simulink model "rotor_simulink"  (R2022a)
settings: Solver=VariableStepAuto  StartTime=0.1  StopTime=60  FixedStep=sample_time/10  RelTol=1e-3
values from neighbouring files (symbols this model uses):
  I_eq = rotor.I + generator.I/gearbox.ratio^2    [parameters.m]
  K_opt = 0.5*(lambda_opt)^(-3)*rho*pi*rotor.R^5*cp_max    [rotor_test.m]
  lambda_vector = linspace(lambda_range(1), lambda_range(2), lambda_item)    [parameters.m]
  omega_rated = rated_values(2)    [parameters.m]
  pitch_range = deg2rad([-15 90])    [parameters.m]
  pitch_vector = linspace(pitch_range(1), pitch_range(2), pitch_item)    [parameters.m]
  rho = 1.225    [parameters.m]
  wind_speed = run_generated_wind_series(wind.mean(i),          wind.turbulence(i), wind_speed, stop_time)    [main.m]    (also in parameters.m = load('usim.dat'); rotor_test.m = WS(i))
undefined symbols (not defined in the file or in its folder): blade, gearbox, generator, lookup_cP, omega_r, rotor
settings Model: Creator=Niccolò  LastModifiedBy=Niccolò

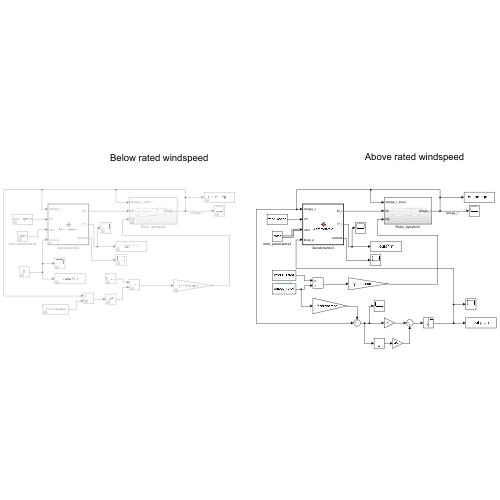
[thumbnail: Simulink's stored preview of the top-level diagram]
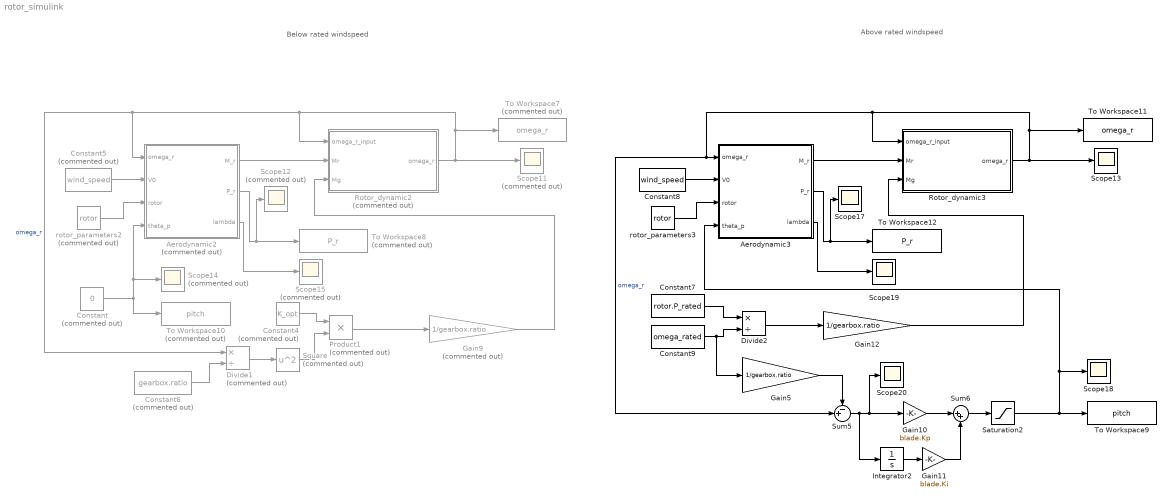
== system rotor_simulink ==
  note: Below rated windspeed
  note: Above rated windspeed
  Aerodynamic2 : MATLAB Function  Commented=on  TreatAsAtomicUnit=on
  Aerodynamic3 : MATLAB Function  TreatAsAtomicUnit=on
  Constant : Constant  Commented=on  Value=0
  Constant4 : Constant  Commented=on  Value=K_opt
  Constant5 : Constant  Commented=on  Value=wind_speed
  Constant6 : Constant  Commented=on  Value=gearbox.ratio
  Constant7 : Constant  Value=rotor.P_rated
  Constant8 : Constant  Value=wind_speed
  Constant9 : Constant  Value=omega_rated
  Divide1 : Product  Commented=on  Inputs=*/
  Divide2 : Product  Inputs=*/
  Gain10 : Gain  Gain=blade.Kp
  Gain11 : Gain  Gain=blade.Ki
  Gain12 : Gain  Gain=1/gearbox.ratio
  Gain5 : Gain  Gain=1/gearbox.ratio
  Gain9 : Gain  Commented=on  Gain=1/gearbox.ratio
  Integrator2 : Integrator
  Product1 : Product  Commented=on
  Rotor_dynamic2 : Subsystem  Commented=on
  Rotor_dynamic3 : Subsystem
  Saturation2 : Saturate  UpperLimit=30*pi/180  LowerLimit=pitch_range(1)
  Scope{11..12,14..15} (4 alike) : Scope  Commented=on
  Scope{13,17..20} (5 alike) : Scope
  Square : Math  Commented=on  Operator=square
  Sum5 : Sum  Inputs=-+|
  Sum6 : Sum  Inputs=|++
  To Workspace10 : ToWorkspace  Commented=on  VariableName=pitch  SaveFormat=Timeseries  SampleTime=-1
  To Workspace11 : ToWorkspace  VariableName=omega_r  SaveFormat=Timeseries  SampleTime=-1
  To Workspace12 : ToWorkspace  VariableName=P_r  SaveFormat=Timeseries  SampleTime=-1
  To Workspace7 : ToWorkspace  Commented=on  VariableName=omega_r  SaveFormat=Timeseries  SampleTime=-1
  To Workspace8 : ToWorkspace  Commented=on  VariableName=P_r  SaveFormat=Timeseries  SampleTime=-1
  To Workspace9 : ToWorkspace  VariableName=pitch  SaveFormat=Timeseries  SampleTime=-1
  rotor_parameters2 : Constant  Commented=on  Value=rotor  OutDataTypeStr=Bus: rotor_bus
  rotor_parameters3 : Constant  Value=rotor  OutDataTypeStr=Bus: rotor_bus
  wires:
  Rotor_dynamic2/1(omega_r) -> Scope11/1, To Workspace7/1, Rotor_dynamic2/1(omega_r_input), Divide1/1, Aerodynamic2/1(omega_r)  "omega_r"
  Constant5/1 -> Aerodynamic2/2(V0)
  Aerodynamic2/2(P_r) -> Scope12/1, To Workspace8/1
  Gain9/1 -> Rotor_dynamic2/3(Mg)
  Aerodynamic2/3(lambda) -> Scope15/1
  Aerodynamic2/1(M_r) -> Rotor_dynamic2/2(Mr)
  rotor_parameters2/1 -> Aerodynamic2/3(rotor)
  Saturation2/1 -> To Workspace9/1, Scope18/1, Aerodynamic3/4(theta_p)
  Sum6/1 -> Saturation2/1
  Constant7/1 -> Divide2/1
  Gain5/1 -> Sum5/1
  rotor_parameters3/1 -> Aerodynamic3/3(rotor)
  Integrator2/1 -> Gain11/1
  Aerodynamic3/1(M_r) -> Rotor_dynamic3/2(Mr)
  Aerodynamic3/3(lambda) -> Scope19/1
  Aerodynamic3/2(P_r) -> Scope17/1, To Workspace12/1
  Divide2/1 -> Gain12/1
  Gain10/1 -> Sum6/1
  Gain12/1 -> Rotor_dynamic3/3(Mg)
  Constant8/1 -> Aerodynamic3/2(V0)
  Constant9/1 -> Gain5/1, Divide2/2
  Sum5/1 -> Scope20/1, Gain10/1, Integrator2/1
  Gain11/1 -> Sum6/2
  Rotor_dynamic3/1(omega_r) -> Scope13/1, To Workspace11/1, Rotor_dynamic3/1(omega_r_input), Sum5/2, Aerodynamic3/1(omega_r)  "omega_r"
  Constant/1 -> Aerodynamic2/4(theta_p), Scope14/1, To Workspace10/1
  Constant4/1 -> Product1/1
  Divide1/1 -> Square/1
  Square/1 -> Product1/2
  Product1/1 -> Gain9/1
  Constant6/1 -> Divide1/2

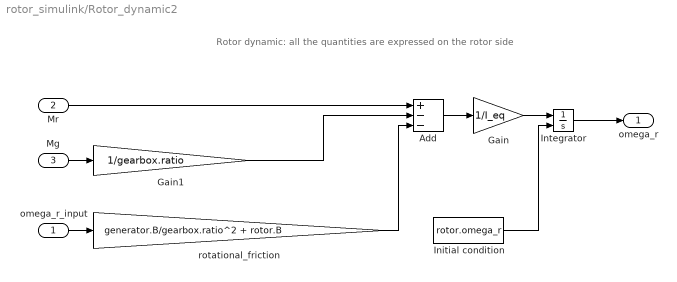
== system rotor_simulink/Rotor_dynamic2 ==
  note: Rotor dynamic: all the quantities are expressed on the rotor side
  omega_r_input : Inport
  Mr : Inport  Port=2
  Mg : Inport  Port=3
  Add : Sum  Inputs=+--
  Gain : Gain  Gain=1/I_eq
  Gain1 : Gain  Gain=1/gearbox.ratio
  Initial condition : Constant  Value=rotor.omega_r
  Integrator : Integrator  InitialConditionSource=external  InitialCondition=omega_r
  rotational_friction : Gain  Gain=generator.B/gearbox.ratio^2 + rotor.B
  omega_r : Outport
  wires:
  Add/1 -> Gain/1
  Gain/1 -> Integrator/1
  Mr/1 -> Add/1
  Initial condition/1 -> Integrator/2
  omega_r_input/1 -> rotational_friction/1
  rotational_friction/1 -> Add/3
  Mg/1 -> Gain1/1
  Gain1/1 -> Add/2
  Integrator/1 -> omega_r/1

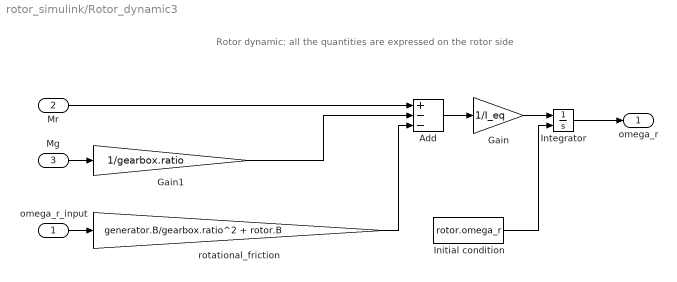
== system rotor_simulink/Rotor_dynamic3 ==
  note: Rotor dynamic: all the quantities are expressed on the rotor side
  omega_r_input : Inport
  Mr : Inport  Port=2
  Mg : Inport  Port=3
  Add : Sum  Inputs=+--
  Gain : Gain  Gain=1/I_eq
  Gain1 : Gain  Gain=1/gearbox.ratio
  Initial condition : Constant  Value=rotor.omega_r
  Integrator : Integrator  InitialConditionSource=external  InitialCondition=omega_r
  rotational_friction : Gain  Gain=generator.B/gearbox.ratio^2 + rotor.B
  omega_r : Outport
  wires:
  Add/1 -> Gain/1
  Gain/1 -> Integrator/1
  Mr/1 -> Add/1
  Initial condition/1 -> Integrator/2
  omega_r_input/1 -> rotational_friction/1
  rotational_friction/1 -> Add/3
  Mg/1 -> Gain1/1
  Gain1/1 -> Add/2
  Integrator/1 -> omega_r/1

== matlab function rotor_simulink/Aerodynamic2 ==
  data: omega_r input; V0 input; M_r output; P_r output; rho parameter; rotor input; theta_p input; lambda_vector parameter; pitch_vector parameter; lookup_cP parameter; lambda output
function [M_r, P_r, lambda] = Aerodynamic(omega_r, V0, rho, rotor, ...
  theta_p, lambda_vector, pitch_vector, lookup_cP) 

R = rotor.R;                  % rotor radius [m]

% retrive the cP from the look-up table
lambda = omega_r*R/V0;                                                
cP = interp2(lambda_vector, pitch_vector, lookup_cP, lambda, theta_p);

P_r = 0.5*rho*V0^3*pi*R^2*cP; % rotor power [W]
M_r = P_r/omega_r;            % rotor torque [Nm]

== matlab function rotor_simulink/Aerodynamic3 ==
  data: omega_r input; V0 input; M_r output; P_r output; rho parameter; rotor input; theta_p input; lambda_vector parameter; pitch_vector parameter; lookup_cP parameter; lambda output
function [M_r, P_r, lambda] = Aerodynamic(omega_r, V0, rho, rotor, ...
  theta_p, lambda_vector, pitch_vector, lookup_cP) 

R = rotor.R;                  % rotor radius [m]

% retrive the cP from the look-up table
lambda = omega_r*R/V0;                                                
cP = interp2(lambda_vector, pitch_vector, lookup_cP, lambda, theta_p);

P_r = 0.5*rho*V0^3*pi*R^2*cP; % rotor power [W]
M_r = P_r/omega_r;            % rotor torque [Nm]
